simulink library "PressureLibrary"  (R2019b)
settings: Solver=VariableStepAuto  StartTime=0.0  StopTime=10.0  RelTol=1e-3
libraries: arduinolib x34, $bdroot x2
settings Model: Creator=staronm3  LastModifiedBy=staronm3

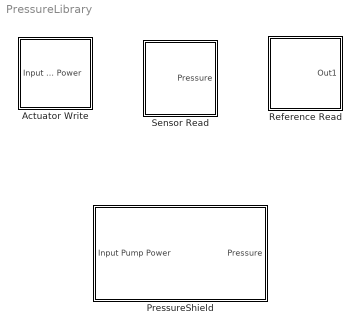
== system PressureLibrary ==
  "Actuator Write " : Subsystem
  "PressureShield " : Subsystem
  Reference Read : Subsystem
  Sensor Read : Subsystem

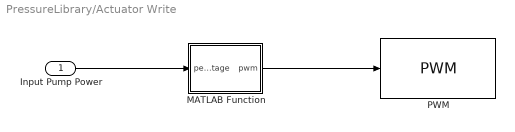
== system PressureLibrary/Actuator Write  ==
  Input Pump Power : Inport
  MATLAB Function : MATLAB Function  TreatAsAtomicUnit=on  SystemSampleTime=0.01
  PWM : arduinolib/PWM  pinNumber=11  EnableInputFrequency=off  InitialFrequency=2000  InitialDutyCycle=0  NotificationType=None  blockPlatform=arduino
  wires:
  Input Pump Power/1 -> MATLAB Function/1(percentage)
  MATLAB Function/1(pwm) -> PWM/1

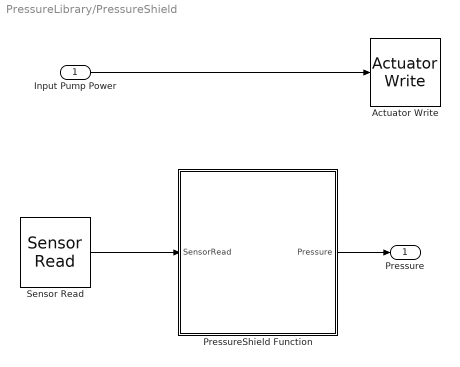
== system PressureLibrary/PressureShield  ==
  "Input Pump Power " : Inport
  "Actuator Write " : $bdroot/Actuator Write   SystemSampleTime=-1  Latency=0  AutoFrameSizeCalculation=off
  PressureShield Function : MATLAB Function  TreatAsAtomicUnit=on  SystemSampleTime=0.1
  Sensor Read : $bdroot/Sensor Read  SystemSampleTime=-1  Latency=0  AutoFrameSizeCalculation=off
  "Pressure " : Outport
  wires:
  "Input Pump Power "/1 -> "Actuator Write "/1
  PressureShield Function/1(Pressure) -> "Pressure "/1
  Sensor Read/1 -> PressureShield Function/1(SensorRead)

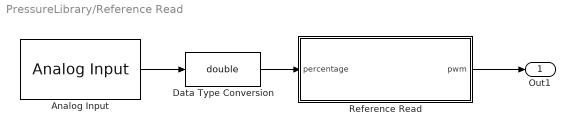
== system PressureLibrary/Reference Read ==
  Analog Input : arduinolib/Analog Input  pinNumber=0  ReadResultsOnly=off  ConversionTriggerSource=Software  ExternalTriggerType=uint32(0)  OutputDataType=uint16  EnableConversionCompleteNotify=off  EnableOuputStatus=off  SampleTime=-1  blockPlatform=arduino
  Data Type Conversion : DataTypeConversion  OutDataTypeStr=double
  Reference Read : MATLAB Function  TreatAsAtomicUnit=on  SystemSampleTime=0.01
  Out1 : Outport
  wires:
  Analog Input/1 -> Data Type Conversion/1
  Reference Read/1(pwm) -> Out1/1
  Data Type Conversion/1 -> Reference Read/1(percentage)

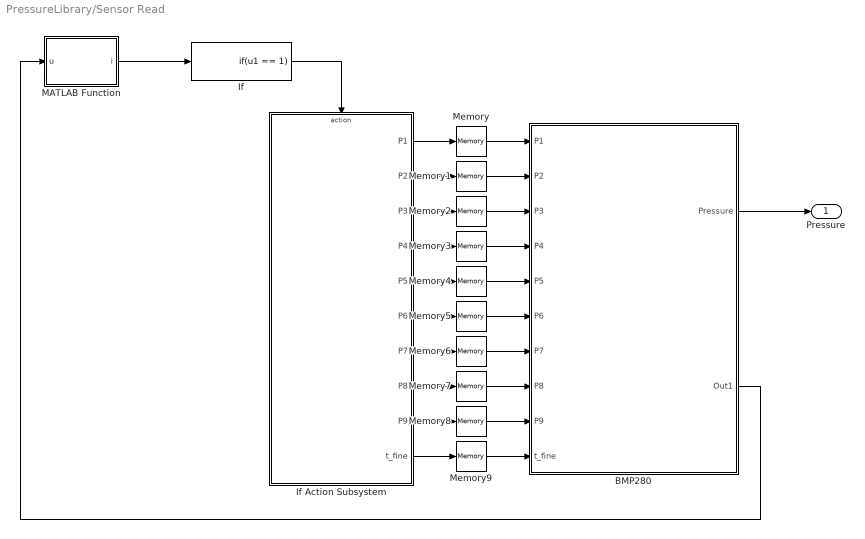
== system PressureLibrary/Sensor Read ==
  "BMP280 " : Subsystem
  If : If  IfExpression=u1 == 1  ShowElse=off
  If Action Subsystem : Subsystem  TreatAsAtomicUnit=on  mask{Ts=0.1}
      mask prompts: Ts "Sampling period (s)"
  MATLAB Function : MATLAB Function  TreatAsAtomicUnit=on  SystemSampleTime=0.1
  Memory{,1..9} (10 alike) : Memory
  Pressure : Outport
  wires:
  If Action Subsystem/1(P1) -> Memory/1
  If Action Subsystem/2(P2) -> Memory1/1
  If Action Subsystem/3(P3) -> Memory2/1
  If Action Subsystem/4(P4) -> Memory3/1
  If Action Subsystem/5(P5) -> Memory4/1
  If Action Subsystem/6(P6) -> Memory5/1
  If Action Subsystem/7(P7) -> Memory6/1
  If Action Subsystem/8(P8) -> Memory7/1
  If Action Subsystem/9(P9) -> Memory8/1
  If Action Subsystem/10(t_fine) -> Memory9/1
  "BMP280 "/1(Pressure) -> Pressure/1
  "BMP280 "/2(Out1) -> MATLAB Function/1(u)
  If/1 -> If Action Subsystem/Action
  MATLAB Function/1(i) -> If/1
  Memory/1 -> "BMP280 "/1(P1)
  Memory1/1 -> "BMP280 "/2(P2)
  Memory2/1 -> "BMP280 "/3(P3)
  Memory3/1 -> "BMP280 "/4(P4)
  Memory4/1 -> "BMP280 "/5(P5)
  Memory5/1 -> "BMP280 "/6(P6)
  Memory6/1 -> "BMP280 "/7(P7)
  Memory7/1 -> "BMP280 "/8(P8)
  Memory8/1 -> "BMP280 "/9(P9)
  Memory9/1 -> "BMP280 "/10(t_fine)

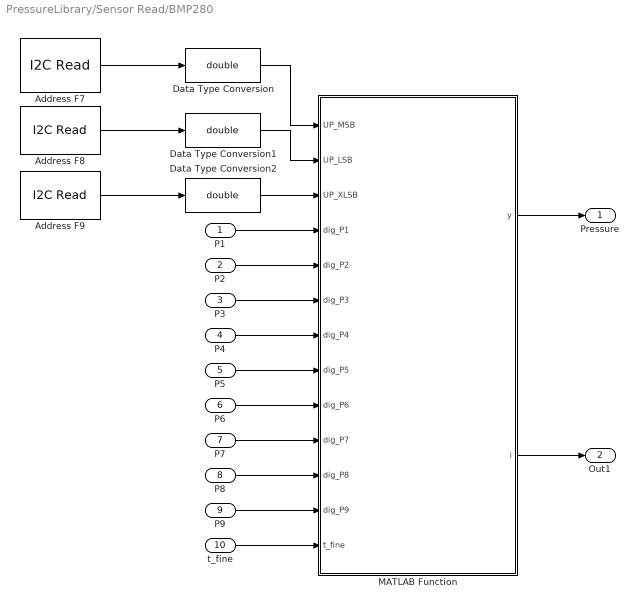
== system PressureLibrary/Sensor Read/BMP280  ==
  P1 : Inport
  P2 : Inport  Port=2
  P3 : Inport  Port=3
  P4 : Inport  Port=4
  P5 : Inport  Port=5
  P6 : Inport  Port=6
  P7 : Inport  Port=7
  P8 : Inport  Port=8
  P9 : Inport  Port=9
  t_fine : Inport  Port=10
  Address F7 : arduinolib/I2C Read  I2CModule=0  Mode=Master  SlaveAddress=118  SlaveByteOrder=BigEndian  Direction=Receiver  RegisterAddressMode=on  RegisterAddress=hex2dec('F7')  SlaveDataType=uint8  DataLength=1  NoAck=off  RepeatedStart=off  OutputStatus=off  blockPlatform=ARDUINO  SampleTime=0.01
      settings: SourceProductName=Simulink Support Package for Arduino Hardware  SourceProductBaseCode=ARDUINO
  Address F8 : arduinolib/I2C Read  I2CModule=0  Mode=Master  SlaveAddress=118  SlaveByteOrder=BigEndian  Direction=Receiver  RegisterAddressMode=on  RegisterAddress=hex2dec('F8')  SlaveDataType=uint8  DataLength=1  NoAck=off  RepeatedStart=off  OutputStatus=off  blockPlatform=ARDUINO  SampleTime=0.01
      settings: SourceProductName=Simulink Support Package for Arduino Hardware  SourceProductBaseCode=ARDUINO
  "Address F9 " : arduinolib/I2C Read  I2CModule=0  Mode=Master  SlaveAddress=118  SlaveByteOrder=BigEndian  Direction=Receiver  RegisterAddressMode=on  RegisterAddress=hex2dec('F9')  SlaveDataType=uint8  DataLength=1  NoAck=off  RepeatedStart=off  OutputStatus=off  blockPlatform=ARDUINO  SampleTime=0.01
      settings: SourceProductName=Simulink Support Package for Arduino Hardware  SourceProductBaseCode=ARDUINO
  Data Type Conversion : DataTypeConversion  OutDataTypeStr=double  ConvertRealWorld=Stored Integer (SI)
  Data Type Conversion1 : DataTypeConversion  OutDataTypeStr=double  ConvertRealWorld=Stored Integer (SI)
  Data Type Conversion2 : DataTypeConversion  OutDataTypeStr=double  ConvertRealWorld=Stored Integer (SI)
  MATLAB Function : MATLAB Function  TreatAsAtomicUnit=on  SystemSampleTime=0.1
  Pressure : Outport
  Out1 : Outport  Port=2
  wires:
  MATLAB Function/1(y) -> Pressure/1
  Address F8/1 -> Data Type Conversion1/1
  "Address F9 "/1 -> Data Type Conversion2/1
  Address F7/1 -> Data Type Conversion/1
  Data Type Conversion/1 -> MATLAB Function/1(UP_MSB)
  Data Type Conversion1/1 -> MATLAB Function/2(UP_LSB)
  Data Type Conversion2/1 -> MATLAB Function/3(UP_XLSB)
  P1/1 -> MATLAB Function/4(dig_P1)
  P2/1 -> MATLAB Function/5(dig_P2)
  P3/1 -> MATLAB Function/6(dig_P3)
  P4/1 -> MATLAB Function/7(dig_P4)
  P5/1 -> MATLAB Function/8(dig_P5)
  P6/1 -> MATLAB Function/9(dig_P6)
  P7/1 -> MATLAB Function/10(dig_P7)
  P8/1 -> MATLAB Function/11(dig_P8)
  P9/1 -> MATLAB Function/12(dig_P9)
  t_fine/1 -> MATLAB Function/13(t_fine)
  MATLAB Function/2(i) -> Out1/1

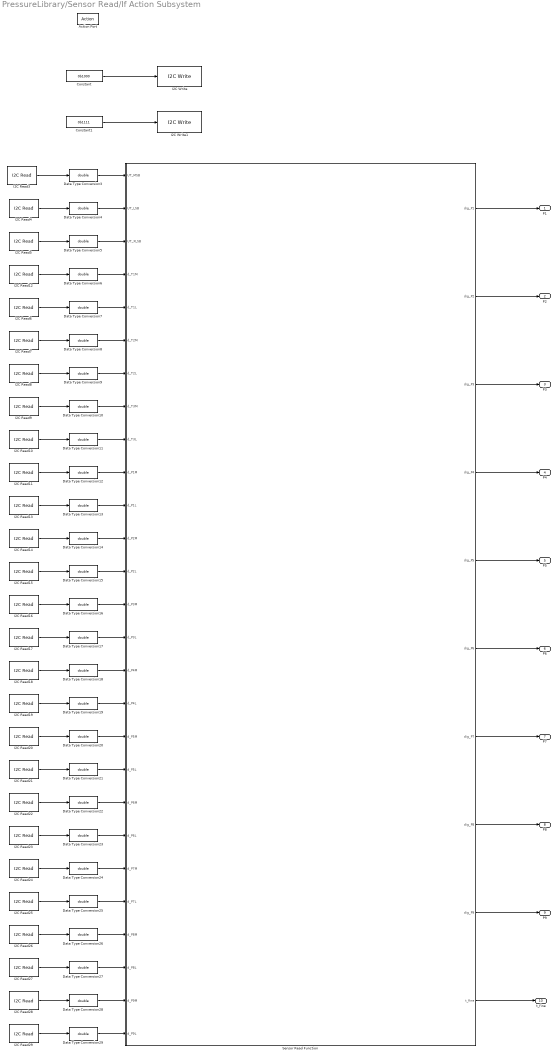
== system PressureLibrary/Sensor Read/If Action Subsystem ==
  Action Port : ActionPort  ActionPortLabel=if(u1 == 1)
  Constant : Constant  Value=0b1000  VectorParams1D=off  OutDataTypeStr=uint8
  Constant1 : Constant  Value=0b1111  OutDataTypeStr=uint8
  Data Type Conversion{3..29} (27 alike) : DataTypeConversion  OutDataTypeStr=double  ConvertRealWorld=Stored Integer (SI)
  I2C Read10 : arduinolib/I2C Read  I2CModule=0  Mode=Master  SlaveAddress=118  SlaveByteOrder=BigEndian  Direction=Receiver  RegisterAddressMode=on  RegisterAddress=hex2dec('8C')  SlaveDataType=uint8  DataLength=1  NoAck=off  RepeatedStart=off  OutputStatus=off  blockPlatform=ARDUINO  SampleTime=Ts
      settings: SourceProductName=Simulink Support Package for Arduino Hardware  SourceProductBaseCode=ARDUINO
  I2C Read11 : arduinolib/I2C Read  I2CModule=0  Mode=Master  SlaveAddress=118  SlaveByteOrder=BigEndian  Direction=Receiver  RegisterAddressMode=on  RegisterAddress=hex2dec('8F')  SlaveDataType=uint8  DataLength=1  NoAck=off  RepeatedStart=off  OutputStatus=off  blockPlatform=ARDUINO  SampleTime=Ts
      settings: SourceProductName=Simulink Support Package for Arduino Hardware  SourceProductBaseCode=ARDUINO
  I2C Read12 : arduinolib/I2C Read  I2CModule=0  Mode=Master  SlaveAddress=118  SlaveByteOrder=BigEndian  Direction=Receiver  RegisterAddressMode=on  RegisterAddress=hex2dec('89')  SlaveDataType=uint8  DataLength=1  NoAck=off  RepeatedStart=off  OutputStatus=off  blockPlatform=ARDUINO  SampleTime=Ts
      settings: SourceProductName=Simulink Support Package for Arduino Hardware  SourceProductBaseCode=ARDUINO
  I2C Read13 : arduinolib/I2C Read  I2CModule=0  Mode=Master  SlaveAddress=118  SlaveByteOrder=BigEndian  Direction=Receiver  RegisterAddressMode=on  RegisterAddress=hex2dec('8E')  SlaveDataType=uint8  DataLength=1  NoAck=off  RepeatedStart=off  OutputStatus=off  blockPlatform=ARDUINO  SampleTime=Ts
      settings: SourceProductName=Simulink Support Package for Arduino Hardware  SourceProductBaseCode=ARDUINO
  I2C Read14 : arduinolib/I2C Read  I2CModule=0  Mode=Master  SlaveAddress=118  SlaveByteOrder=BigEndian  Direction=Receiver  RegisterAddressMode=on  RegisterAddress=hex2dec('91')  SlaveDataType=uint8  DataLength=1  NoAck=off  RepeatedStart=off  OutputStatus=off  blockPlatform=ARDUINO  SampleTime=Ts
      settings: SourceProductName=Simulink Support Package for Arduino Hardware  SourceProductBaseCode=ARDUINO
  I2C Read15 : arduinolib/I2C Read  I2CModule=0  Mode=Master  SlaveAddress=118  SlaveByteOrder=BigEndian  Direction=Receiver  RegisterAddressMode=on  RegisterAddress=hex2dec('90')  SlaveDataType=uint8  DataLength=1  NoAck=off  RepeatedStart=off  OutputStatus=off  blockPlatform=ARDUINO  SampleTime=Ts
      settings: SourceProductName=Simulink Support Package for Arduino Hardware  SourceProductBaseCode=ARDUINO
  I2C Read16 : arduinolib/I2C Read  I2CModule=0  Mode=Master  SlaveAddress=118  SlaveByteOrder=BigEndian  Direction=Receiver  RegisterAddressMode=on  RegisterAddress=hex2dec('93')  SlaveDataType=uint8  DataLength=1  NoAck=off  RepeatedStart=off  OutputStatus=off  blockPlatform=ARDUINO  SampleTime=Ts
      settings: SourceProductName=Simulink Support Package for Arduino Hardware  SourceProductBaseCode=ARDUINO
  I2C Read17 : arduinolib/I2C Read  I2CModule=0  Mode=Master  SlaveAddress=118  SlaveByteOrder=BigEndian  Direction=Receiver  RegisterAddressMode=on  RegisterAddress=hex2dec('92')  SlaveDataType=uint8  DataLength=1  NoAck=off  RepeatedStart=off  OutputStatus=off  blockPlatform=ARDUINO  SampleTime=Ts
      settings: SourceProductName=Simulink Support Package for Arduino Hardware  SourceProductBaseCode=ARDUINO
  I2C Read18 : arduinolib/I2C Read  I2CModule=0  Mode=Master  SlaveAddress=118  SlaveByteOrder=BigEndian  Direction=Receiver  RegisterAddressMode=on  RegisterAddress=hex2dec('95')  SlaveDataType=uint8  DataLength=1  NoAck=off  RepeatedStart=off  OutputStatus=off  blockPlatform=ARDUINO  SampleTime=Ts
      settings: SourceProductName=Simulink Support Package for Arduino Hardware  SourceProductBaseCode=ARDUINO
  I2C Read19 : arduinolib/I2C Read  I2CModule=0  Mode=Master  SlaveAddress=118  SlaveByteOrder=BigEndian  Direction=Receiver  RegisterAddressMode=on  RegisterAddress=hex2dec('94')  SlaveDataType=uint8  DataLength=1  NoAck=off  RepeatedStart=off  OutputStatus=off  blockPlatform=ARDUINO  SampleTime=Ts
      settings: SourceProductName=Simulink Support Package for Arduino Hardware  SourceProductBaseCode=ARDUINO
  I2C Read20 : arduinolib/I2C Read  I2CModule=0  Mode=Master  SlaveAddress=118  SlaveByteOrder=BigEndian  Direction=Receiver  RegisterAddressMode=on  RegisterAddress=hex2dec('97')  SlaveDataType=uint8  DataLength=1  NoAck=off  RepeatedStart=off  OutputStatus=off  blockPlatform=ARDUINO  SampleTime=Ts
      settings: SourceProductName=Simulink Support Package for Arduino Hardware  SourceProductBaseCode=ARDUINO
  I2C Read21 : arduinolib/I2C Read  I2CModule=0  Mode=Master  SlaveAddress=118  SlaveByteOrder=BigEndian  Direction=Receiver  RegisterAddressMode=on  RegisterAddress=hex2dec('96')  SlaveDataType=uint8  DataLength=1  NoAck=off  RepeatedStart=off  OutputStatus=off  blockPlatform=ARDUINO  SampleTime=Ts
      settings: SourceProductName=Simulink Support Package for Arduino Hardware  SourceProductBaseCode=ARDUINO
  I2C Read22 : arduinolib/I2C Read  I2CModule=0  Mode=Master  SlaveAddress=118  SlaveByteOrder=BigEndian  Direction=Receiver  RegisterAddressMode=on  RegisterAddress=hex2dec('99')  SlaveDataType=uint8  DataLength=1  NoAck=off  RepeatedStart=off  OutputStatus=off  blockPlatform=ARDUINO  SampleTime=Ts
      settings: SourceProductName=Simulink Support Package for Arduino Hardware  SourceProductBaseCode=ARDUINO
  I2C Read23 : arduinolib/I2C Read  I2CModule=0  Mode=Master  SlaveAddress=118  SlaveByteOrder=BigEndian  Direction=Receiver  RegisterAddressMode=on  RegisterAddress=hex2dec('98')  SlaveDataType=uint8  DataLength=1  NoAck=off  RepeatedStart=off  OutputStatus=off  blockPlatform=ARDUINO  SampleTime=Ts
      settings: SourceProductName=Simulink Support Package for Arduino Hardware  SourceProductBaseCode=ARDUINO
  I2C Read24 : arduinolib/I2C Read  I2CModule=0  Mode=Master  SlaveAddress=118  SlaveByteOrder=BigEndian  Direction=Receiver  RegisterAddressMode=on  RegisterAddress=hex2dec('9B')  SlaveDataType=uint8  DataLength=1  NoAck=off  RepeatedStart=off  OutputStatus=off  blockPlatform=ARDUINO  SampleTime=Ts
      settings: SourceProductName=Simulink Support Package for Arduino Hardware  SourceProductBaseCode=ARDUINO
  I2C Read25 : arduinolib/I2C Read  I2CModule=0  Mode=Master  SlaveAddress=118  SlaveByteOrder=BigEndian  Direction=Receiver  RegisterAddressMode=on  RegisterAddress=hex2dec('9A')  SlaveDataType=uint8  DataLength=1  NoAck=off  RepeatedStart=off  OutputStatus=off  blockPlatform=ARDUINO  SampleTime=Ts
      settings: SourceProductName=Simulink Support Package for Arduino Hardware  SourceProductBaseCode=ARDUINO
  I2C Read26 : arduinolib/I2C Read  I2CModule=0  Mode=Master  SlaveAddress=118  SlaveByteOrder=BigEndian  Direction=Receiver  RegisterAddressMode=on  RegisterAddress=hex2dec('9D')  SlaveDataType=uint8  DataLength=1  NoAck=off  RepeatedStart=off  OutputStatus=off  blockPlatform=ARDUINO  SampleTime=Ts
      settings: SourceProductName=Simulink Support Package for Arduino Hardware  SourceProductBaseCode=ARDUINO
  I2C Read27 : arduinolib/I2C Read  I2CModule=0  Mode=Master  SlaveAddress=118  SlaveByteOrder=BigEndian  Direction=Receiver  RegisterAddressMode=on  RegisterAddress=hex2dec('9C')  SlaveDataType=uint8  DataLength=1  NoAck=off  RepeatedStart=off  OutputStatus=off  blockPlatform=ARDUINO  SampleTime=Ts
      settings: SourceProductName=Simulink Support Package for Arduino Hardware  SourceProductBaseCode=ARDUINO
  I2C Read28 : arduinolib/I2C Read  I2CModule=0  Mode=Master  SlaveAddress=118  SlaveByteOrder=BigEndian  Direction=Receiver  RegisterAddressMode=on  RegisterAddress=hex2dec('9F')  SlaveDataType=uint8  DataLength=1  NoAck=off  RepeatedStart=off  OutputStatus=off  blockPlatform=ARDUINO  SampleTime=Ts
      settings: SourceProductName=Simulink Support Package for Arduino Hardware  SourceProductBaseCode=ARDUINO
  I2C Read29 : arduinolib/I2C Read  I2CModule=0  Mode=Master  SlaveAddress=118  SlaveByteOrder=BigEndian  Direction=Receiver  RegisterAddressMode=on  RegisterAddress=hex2dec('9E')  SlaveDataType=uint8  DataLength=1  NoAck=off  RepeatedStart=off  OutputStatus=off  blockPlatform=ARDUINO  SampleTime=Ts
      settings: SourceProductName=Simulink Support Package for Arduino Hardware  SourceProductBaseCode=ARDUINO
  I2C Read3 : arduinolib/I2C Read  I2CModule=0  Mode=Master  SlaveAddress=118  SlaveByteOrder=BigEndian  Direction=Receiver  RegisterAddressMode=on  RegisterAddress=hex2dec('FA')  SlaveDataType=uint8  DataLength=1  NoAck=off  RepeatedStart=off  OutputStatus=off  blockPlatform=ARDUINO  SampleTime=Ts
      settings: SourceProductName=Simulink Support Package for Arduino Hardware  SourceProductBaseCode=ARDUINO
  I2C Read4 : arduinolib/I2C Read  I2CModule=0  Mode=Master  SlaveAddress=118  SlaveByteOrder=BigEndian  Direction=Receiver  RegisterAddressMode=on  RegisterAddress=hex2dec('FB')  SlaveDataType=uint8  DataLength=1  NoAck=off  RepeatedStart=off  OutputStatus=off  blockPlatform=ARDUINO  SampleTime=Ts
      settings: SourceProductName=Simulink Support Package for Arduino Hardware  SourceProductBaseCode=ARDUINO
  I2C Read5 : arduinolib/I2C Read  I2CModule=0  Mode=Master  SlaveAddress=118  SlaveByteOrder=BigEndian  Direction=Receiver  RegisterAddressMode=on  RegisterAddress=hex2dec('FC')  SlaveDataType=uint8  DataLength=1  NoAck=off  RepeatedStart=off  OutputStatus=off  blockPlatform=ARDUINO  SampleTime=Ts
      settings: SourceProductName=Simulink Support Package for Arduino Hardware  SourceProductBaseCode=ARDUINO
  I2C Read6 : arduinolib/I2C Read  I2CModule=0  Mode=Master  SlaveAddress=118  SlaveByteOrder=BigEndian  Direction=Receiver  RegisterAddressMode=on  RegisterAddress=hex2dec('88')  SlaveDataType=uint8  DataLength=1  NoAck=off  RepeatedStart=off  OutputStatus=off  blockPlatform=ARDUINO  SampleTime=Ts
      settings: SourceProductName=Simulink Support Package for Arduino Hardware  SourceProductBaseCode=ARDUINO
  I2C Read7 : arduinolib/I2C Read  I2CModule=0  Mode=Master  SlaveAddress=118  SlaveByteOrder=BigEndian  Direction=Receiver  RegisterAddressMode=on  RegisterAddress=hex2dec('8B')  SlaveDataType=uint8  DataLength=1  NoAck=off  RepeatedStart=off  OutputStatus=off  blockPlatform=ARDUINO  SampleTime=Ts
      settings: SourceProductName=Simulink Support Package for Arduino Hardware  SourceProductBaseCode=ARDUINO
  I2C Read8 : arduinolib/I2C Read  I2CModule=0  Mode=Master  SlaveAddress=118  SlaveByteOrder=BigEndian  Direction=Receiver  RegisterAddressMode=on  RegisterAddress=hex2dec('8A')  SlaveDataType=uint8  DataLength=1  NoAck=off  RepeatedStart=off  OutputStatus=off  blockPlatform=ARDUINO  SampleTime=Ts
      settings: SourceProductName=Simulink Support Package for Arduino Hardware  SourceProductBaseCode=ARDUINO
  I2C Read9 : arduinolib/I2C Read  I2CModule=0  Mode=Master  SlaveAddress=118  SlaveByteOrder=BigEndian  Direction=Receiver  RegisterAddressMode=on  RegisterAddress=hex2dec('8D')  SlaveDataType=uint8  DataLength=1  NoAck=off  RepeatedStart=off  OutputStatus=off  blockPlatform=ARDUINO  SampleTime=Ts
      settings: SourceProductName=Simulink Support Package for Arduino Hardware  SourceProductBaseCode=ARDUINO
  I2C Write : arduinolib/I2C Write  I2CModule=0  Mode=Master  SlaveAddress=118  SlaveByteOrder=LittleEndian  Direction=Transmitter  RegisterAddressMode=on  RegisterAddress=hex2dec('F5')  SlaveDataType=uint8  DataLength=1  NoAck=off  RepeatedStart=off  OutputStatus=off  blockPlatform=ARDUINO
      settings: SourceProductName=Simulink Support Package for Arduino Hardware  SourceProductBaseCode=ARDUINO
  I2C Write1 : arduinolib/I2C Write  I2CModule=0  Mode=Master  SlaveAddress=118  SlaveByteOrder=LittleEndian  Direction=Transmitter  RegisterAddressMode=on  RegisterAddress=hex2dec('F4')  SlaveDataType=uint8  DataLength=1  NoAck=off  RepeatedStart=off  OutputStatus=off  blockPlatform=ARDUINO
      settings: SourceProductName=Simulink Support Package for Arduino Hardware  SourceProductBaseCode=ARDUINO
  Sensor Read Function : MATLAB Function  TreatAsAtomicUnit=on  SystemSampleTime=0.1
  P1 : Outport
  P2 : Outport  Port=2
  P3 : Outport  Port=3
  P4 : Outport  Port=4
  P5 : Outport  Port=5
  P6 : Outport  Port=6
  P7 : Outport  Port=7
  P8 : Outport  Port=8
  P9 : Outport  Port=9
  t_fine : Outport  Port=10
  wires:
  Data Type Conversion20/1 -> Sensor Read Function/18(d_P5M)
  Data Type Conversion4/1 -> Sensor Read Function/2(UT_LSB)
  I2C Read13/1 -> Data Type Conversion13/1
  Sensor Read Function/9(dig_P9) -> P9/1
  Data Type Conversion26/1 -> Sensor Read Function/24(d_P8M)
  I2C Read29/1 -> Data Type Conversion29/1
  Data Type Conversion13/1 -> Sensor Read Function/11(d_P1L)
  Data Type Conversion10/1 -> Sensor Read Function/8(d_T3M)
  I2C Read10/1 -> Data Type Conversion11/1
  I2C Read28/1 -> Data Type Conversion28/1
  Data Type Conversion6/1 -> Sensor Read Function/4(d_T1M)
  Data Type Conversion28/1 -> Sensor Read Function/26(d_P9M)
  Data Type Conversion17/1 -> Sensor Read Function/15(d_P3L)
  I2C Read8/1 -> Data Type Conversion9/1
  Data Type Conversion25/1 -> Sensor Read Function/23(d_P7L)
  Sensor Read Function/1(dig_P1) -> P1/1
  Sensor Read Function/4(dig_P4) -> P4/1
  I2C Read26/1 -> Data Type Conversion26/1
  I2C Read18/1 -> Data Type Conversion18/1
  I2C Read11/1 -> Data Type Conversion12/1
  I2C Read14/1 -> Data Type Conversion14/1
  I2C Read9/1 -> Data Type Conversion10/1
  Data Type Conversion29/1 -> Sensor Read Function/27(d_P9L)
  I2C Read19/1 -> Data Type Conversion19/1
  Sensor Read Function/10(t_fine) -> t_fine/1
  Data Type Conversion19/1 -> Sensor Read Function/17(d_P4L)
  I2C Read12/1 -> Data Type Conversion6/1
  I2C Read6/1 -> Data Type Conversion7/1
  Data Type Conversion14/1 -> Sensor Read Function/12(d_P2M)
  I2C Read25/1 -> Data Type Conversion25/1
  I2C Read20/1 -> Data Type Conversion20/1
  I2C Read5/1 -> Data Type Conversion5/1
  I2C Read15/1 -> Data Type Conversion15/1
  Sensor Read Function/7(dig_P7) -> P7/1
  I2C Read27/1 -> Data Type Conversion27/1
  I2C Read17/1 -> Data Type Conversion17/1
  I2C Read21/1 -> Data Type Conversion21/1
  Data Type Conversion18/1 -> Sensor Read Function/16(d_P4M)
  Data Type Conversion7/1 -> Sensor Read Function/5(d_T1L)
  I2C Read22/1 -> Data Type Conversion22/1
  I2C Read3/1 -> Data Type Conversion3/1
  I2C Read23/1 -> Data Type Conversion23/1
  Constant1/1 -> I2C Write1/1
  Data Type Conversion24/1 -> Sensor Read Function/22(d_P7M)
  Sensor Read Function/3(dig_P3) -> P3/1
  Data Type Conversion9/1 -> Sensor Read Function/7(d_T2L)
  Data Type Conversion3/1 -> Sensor Read Function/1(UT_MSB)
  Data Type Conversion15/1 -> Sensor Read Function/13(d_P2L)
  Data Type Conversion8/1 -> Sensor Read Function/6(d_T2M)
  Data Type Conversion11/1 -> Sensor Read Function/9(d_T3L)
  Data Type Conversion12/1 -> Sensor Read Function/10(d_P1M)
  Data Type Conversion5/1 -> Sensor Read Function/3(UT_XLSB)
  I2C Read24/1 -> Data Type Conversion24/1
  Constant/1 -> I2C Write/1
  Sensor Read Function/2(dig_P2) -> P2/1
  Data Type Conversion27/1 -> Sensor Read Function/25(d_P8L)
  Data Type Conversion23/1 -> Sensor Read Function/21(d_P6L)
  I2C Read7/1 -> Data Type Conversion8/1
  Sensor Read Function/8(dig_P8) -> P8/1
  I2C Read16/1 -> Data Type Conversion16/1
  Data Type Conversion16/1 -> Sensor Read Function/14(d_P3M)
  Data Type Conversion22/1 -> Sensor Read Function/20(d_P6M)
  Sensor Read Function/6(dig_P6) -> P6/1
  Data Type Conversion21/1 -> Sensor Read Function/19(d_P5L)
  I2C Read4/1 -> Data Type Conversion4/1
  Sensor Read Function/5(dig_P5) -> P5/1

== matlab function PressureLibrary/Reference Read/Reference Read ==
  data: percentage input; pwm output
function pwm = fcn(percentage)

pwm = constrain((percentage/10.23), 0, 100);

end

== matlab function PressureLibrary/PressureShield /PressureShield Function ==
  data: SensorRead input; Pressure output
function Pressure = PressureShieldPID(SensorRead)

minVal = 0;
maxVal = 100;

persistent ref;

if isempty(ref) 
tic
while(1)
toc
ref = SensorRead
if (toc>10)
    break;
end 
end
end
Pressure = double((SensorRead-ref)/100);

end

== matlab function PressureLibrary/Actuator Write /MATLAB Function ==
  data: percentage input; pwm output
function pwm = fcn(percentage)

pwm = constrain((percentage * 2.55), 0, 255);

end

== matlab function PressureLibrary/Sensor Read/BMP280 /MATLAB Function ==
  data: UP_MSB input; UP_LSB input; UP_XLSB input; dig_P1 input; y output; dig_P2 input; dig_P3 input; dig_P4 input; dig_P5 input; dig_P6 input; dig_P7 input; dig_P8 input; dig_P9 input; t_fine input; i output
function [y,i]= BMP280(UP_MSB, UP_LSB, UP_XLSB, dig_P1, dig_P2, dig_P3, dig_P4, dig_P5, dig_P6, dig_P7, dig_P8, dig_P9, t_fine)


            UP_MSBbit = bitget(UP_MSB,8:-1:1);
            UP_LSBbit = bitget(UP_LSB,8:-1:1);
            UP_XLSBbit = bitget(UP_XLSB,8:-1:5);
            bitsP = [UP_MSBbit UP_LSBbit UP_XLSBbit];
            adc_p = bi2de(bitsP,'left-msb');
           
            var1 = (t_fine/2)-64000;
            var2 = var1*var1*dig_P6/32768;
            var2 = var2+var1*dig_P5*2;
            var2 = (var2/4)+(dig_P4*65536);
            var1 = (dig_P3*var1*var1/524288+dig_P2*var1)/524288;
            var1 = (1+var1/32768)*dig_P1;
            p = 1048576-adc_p;
            p = (p-(var2/4096))*6250/var1;
            var1 = dig_P9*p*p/2147483648;
            var2 = p*dig_P8/32768;
            y = int32((p+(var1+var2+dig_P7)/16))
            i = 2;
end

== matlab function PressureLibrary/Sensor Read/MATLAB Function ==
  data: u input; i output
function i = fcn(u)

if (isempty(u))
i = 1;
else  
i = 1;
end

end

== matlab function PressureLibrary/Sensor Read/If Action Subsystem/Sensor Read Function ==
  data: UT_MSB input; UT_LSB input; UT_XLSB input; dig_P1 output; d_T1M input; d_T1L input; d_T2M input; d_T2L input; d_T3M input; d_T3L input; d_P1M input; d_P1L input; d_P2M input; d_P2L input; d_P3M input; d_P3L input; d_P4M input; d_P4L input; d_P5M input; d_P5L input; d_P6M input; d_P6L input; d_P7M input; d_P7L input; d_P8M input; d_P8L input; d_P9M input; d_P9L input; dig_P2 output; dig_P3 output; dig_P4 output; dig_P5 output; dig_P6 output; dig_P7 output; dig_P8 output; dig_P9 output; t_fine output
function [dig_P1, dig_P2, dig_P3, dig_P4, dig_P5, dig_P6, dig_P7, dig_P8, dig_P9, t_fine] = BMP280Init(UT_MSB,UT_LSB,UT_XLSB,d_T1M,d_T1L,d_T2M,d_T2L,d_T3M,d_T3L,...
                     d_P1M,d_P1L,d_P2M,d_P2L,d_P3M,d_P3L,d_P4M,d_P4L,d_P5M,d_P5L,d_P6M,d_P6L,d_P7M,d_P7L,...
                     d_P8M,d_P8L,d_P9M,d_P9L)
            
              UT_MSBbit = bitget(UT_MSB,8:-1:1);  
              UT_LSBbit = bitget(UT_LSB,8:-1:1);
              UT_XLSBbit = bitget(UT_XLSB,8:-1:5);
              bitsT = [UT_MSBbit UT_LSBbit UT_XLSBbit];
              adc_t = bi2de(bitsT,'left-msb');
             
              dig_T1Mbit = bitget(d_T1M,8:-1:1);
              dig_T1Lbit = bitget(d_T1L,8:-1:1);
              bitsT1 = [dig_T1Mbit dig_T1Lbit]
              dig_T1 = bi2de(bitsT1,'left-msb');

              dig_T2Mbit = bitget(d_T2M,8:-1:1);
              dig_T2Lbit = bitget(d_T2L,8:-1:1);
              bitsT2 = [dig_T2Mbit dig_T2Lbit]
              dig_T2 = bi2de(bitsT2,'left-msb');
            
              dig_T3Mbit = bitget(d_T3M,8:-1:1);
              dig_T3Lbit = bitget(d_T3L,8:-1:1);
              bitsT3 = [dig_T3Mbit dig_T3Lbit]
              dig_T3 = bi2de(bitsT3,'left-msb');
           
            
              dig_P1Mbit = bitget(d_P1M,8:-1:1);
              dig_P1Lbit = bitget(d_P1L,8:-1:1);
              bitsP1 = [dig_P1Mbit dig_P1Lbit];
              dig_P1 = bi2de(bitsP1,'left-msb');
              
              dig_P2Mbit = bitget(d_P2M,8:-1:1);
              dig_P2Lbit = bitget(d_P2L,8:-1:1);
              bitsP2 = [dig_P2Mbit dig_P2Lbit];
              dig_P2 = bi2de(bitsP2,'left-msb');
              
              dig_P3Mbit = bitget(d_P3M,8:-1:1);
              dig_P3Lbit = bitget(d_P3L,8:-1:1);
              bitsP3 = [dig_P3Mbit dig_P3Lbit];
              dig_P3 = bi2de(bitsP3,'left-msb');
              
              dig_P4Mbit = bitget(d_P4M,8:-1:1);
              dig_P4Lbit = bitget(d_P4L,8:-1:1);
              bitsP4 = [dig_P4Mbit dig_P4Lbit];
              dig_P4 = bi2de(bitsP4,'left-msb');
              
              dig_P5Mbit = bitget(d_P5M,8:-1:1);
              dig_P5Lbit = bitget(d_P5L,8:-1:1);
              bitsP5 = [dig_P5Mbit dig_P5Lbit];
              dig_P5 = bi2de(bitsP5,'left-msb');
              
              dig_P6Mbit = bitget(d_P6M,8:-1:1);
              dig_P6Lbit = bitget(d_P6L,8:-1:1);
              bitsP6 = [dig_P6Mbit dig_P6Lbit];
              dig_P6 = bi2de(bitsP6,'left-msb');
              
              dig_P7Mbit = bitget(d_P7M,8:-1:1);
              dig_P7Lbit = bitget(d_P7L,8:-1:1);
              bitsP7 = [dig_P7Mbit dig_P7Lbit];
              dig_P7 = bi2de(bitsP7,'left-msb');
              
              dig_P8Mbit = bitget(d_P8M,8:-1:1);
              dig_P8Lbit = bitget(d_P8L,8:-1:1);
              bitsP8 = [dig_P8Mbit dig_P8Lbit];
              dig_P8 = bi2de(bitsP8,'left-msb');
              
              dig_P9Mbit = bitget(d_P9M,8:-1:1);
              dig_P9Lbit = bitget(d_P9L,8:-1:1);
              bitsP9 = [dig_P9Mbit dig_P9Lbit];
              dig_P9 = bi2de(bitsP9,'left-msb');

              
            var_1 = ((adc_t)/16384-(dig_T1)/1024)*(dig_T2);
            var_2 = (((adc_t)/131072-(dig_T1)/8192)*((adc_t)/131072-(dig_T1)/8192))*(dig_T3);
            t_fine = var_1 + var_2;
end
